simulink model "simulink1"  (R2020b)
settings: Solver=VariableStepAuto  StartTime=0.0  StopTime=30  RelTol=1e-3
settings Model: Creator=akku  LastModifiedBy=akku

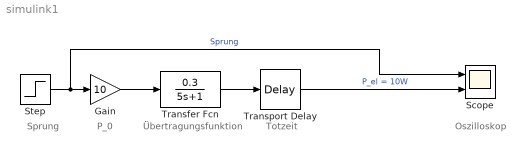
== system simulink1 ==
  note: Oszilloskop
  note: Totzeit
  note: Übertragungsfunktion
  note: P_0
  note: Sprung
  Gain : Gain  Gain=10
  Scope : Scope  NumInputPorts=2
  Step : Step  Time=0  SampleTime=0
  Transfer Fcn : TransferFcn  Numerator=[0.3]  Denominator=[5 1]
  Transport Delay : TransportDelay
  wires:
  Step/1 -> Scope/1, Gain/1  "Sprung"
  Transport Delay/1 -> Scope/2  "P_el = 10W"
  Gain/1 -> Transfer Fcn/1
  Transfer Fcn/1 -> Transport Delay/1
